simulink model "voitureAuto"  (R2019a)
settings: Solver=VariableStepAuto  StartTime=0.0  StopTime=5000  RelTol=1e-3
undefined symbols (not defined in the file or in its folder): BAT_AUTONOMY_KM, INIT_NIV_BAT, TIME_TO_CHARGE_S, VITESSE_MAX_KMH
libraries: simulink x2, simulink_extras x1, truetime x1
settings Model: SimulationMode=accelerator  Creator=PolyMTL  LastModifiedBy=angodb
settings DataIOCC: ReturnWorkspaceOutputs=off
settings OptimizationCC: EfficientMapNaN2IntZero=off
settings DebuggingCC: PregeneratedLibrarySubsystemCodeDiagnostic=none  ArithmeticOperatorsInVariantConditions=warning
settings HardwareCC: TargetBitPerPointer=64  TargetBitPerSizeT=64  TargetBitPerPtrDiffT=64  TargetLongLongMode=on  TargetIntDivRoundTo=Zero  TargetEndianess=LittleEndian  TargetWordSize=64  TargetHWDeviceType=MATLAB Host  ProdEqTarget=off
settings SFSimCC: SimUseLocalCustomCode=off
settings RTWCC: RTWUseLocalCustomCode=off
settings CodeAppCC: MaxIdLength=128
settings GRTTargetCC: TargetLangStandard=C89/C90 (ANSI)  CombineOutputUpdateFcns=off  GRTInterface=on

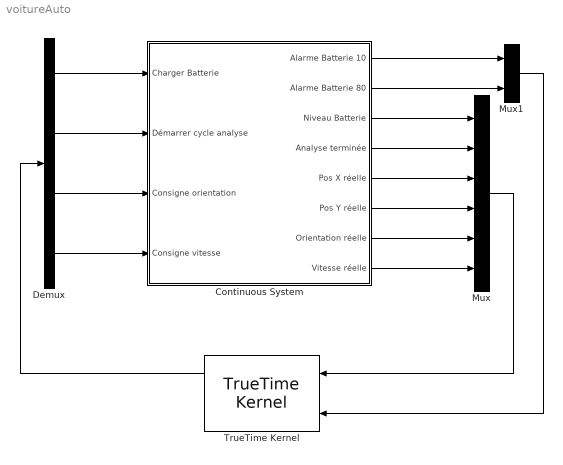
== system voitureAuto ==
  Continuous System : Subsystem
  Demux : Demux
  Mux : Mux  Inputs=6
  Mux1 : Mux  Inputs=2
  TrueTime Kernel : truetime/TrueTime Kernel  sfun=ctrlauto  args=[]  ninputsoutputs=[6 4]  ntriggers=2  trigtype=falling  nwnodenbr=[]  clockoffsetdrift=[0 0]  schedoutput=on  battery=off  poweroutput=off
  wires:
  Continuous System/5(Pos X réelle) -> Mux/3
  Continuous System/4(Analyse terminée) -> Mux/2
  Continuous System/3(Niveau Batterie) -> Mux/1
  Continuous System/8(Vitesse réelle) -> Mux/6
  Continuous System/7(Orientation réelle) -> Mux/5
  Continuous System/6(Pos Y réelle) -> Mux/4
  Demux/1 -> Continuous System/1(Charger Batterie)
  Demux/4 -> Continuous System/4(Consigne vitesse)
  Demux/3 -> Continuous System/3(Consigne orientation)
  Demux/2 -> Continuous System/2(Démarrer cycle analyse)
  Continuous System/1(Alarme Batterie 10) -> Mux1/1
  Continuous System/2(Alarme Batterie 80) -> Mux1/2
  Mux/1 -> TrueTime Kernel/1
  TrueTime Kernel/1 -> Demux/1
  Mux1/1 -> TrueTime Kernel/2

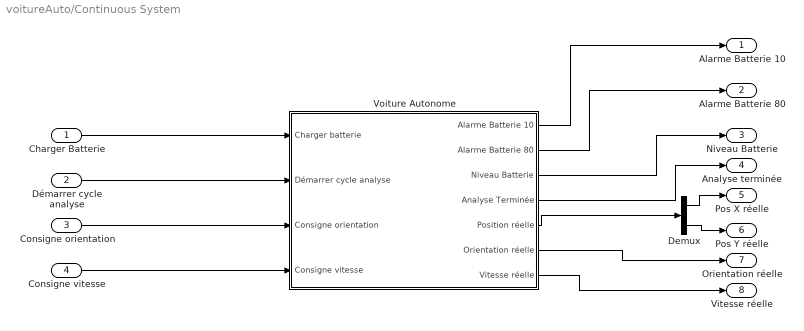
== system voitureAuto/Continuous System ==
  Charger Batterie : Inport
  Démarrer cycle analyse : Inport  Port=2
  Consigne orientation : Inport  Port=3
  Consigne vitesse : Inport  Port=4
  Demux : Demux  Outputs=2
  Voiture Autonome : Subsystem
  Alarme Batterie 10 : Outport
  Alarme Batterie 80 : Outport  Port=2
  Niveau Batterie : Outport  Port=3
  Analyse terminée : Outport  Port=4
  Pos X réelle : Outport  Port=5
  Pos Y réelle : Outport  Port=6
  Orientation réelle : Outport  Port=7
  Vitesse réelle : Outport  Port=8
  wires:
  Consigne orientation/1 -> Voiture Autonome/3(Consigne orientation)
  Démarrer cycle analyse/1 -> Voiture Autonome/2(Démarrer cycle analyse)
  Consigne vitesse/1 -> Voiture Autonome/4(Consigne vitesse)
  Voiture Autonome/3(Niveau Batterie) -> Niveau Batterie/1
  Voiture Autonome/1(Alarme Batterie 10) -> Alarme Batterie 10/1
  Voiture Autonome/4(Analyse Terminée) -> Analyse terminée/1
  Voiture Autonome/6(Orientation réelle) -> Orientation réelle/1
  Voiture Autonome/7(Vitesse réelle) -> Vitesse réelle/1
  Voiture Autonome/5(Position réelle) -> Demux/1
  Demux/1 -> Pos X réelle/1
  Demux/2 -> Pos Y réelle/1
  Charger Batterie/1 -> Voiture Autonome/1(Charger batterie)
  Voiture Autonome/2(Alarme Batterie 80) -> Alarme Batterie 80/1

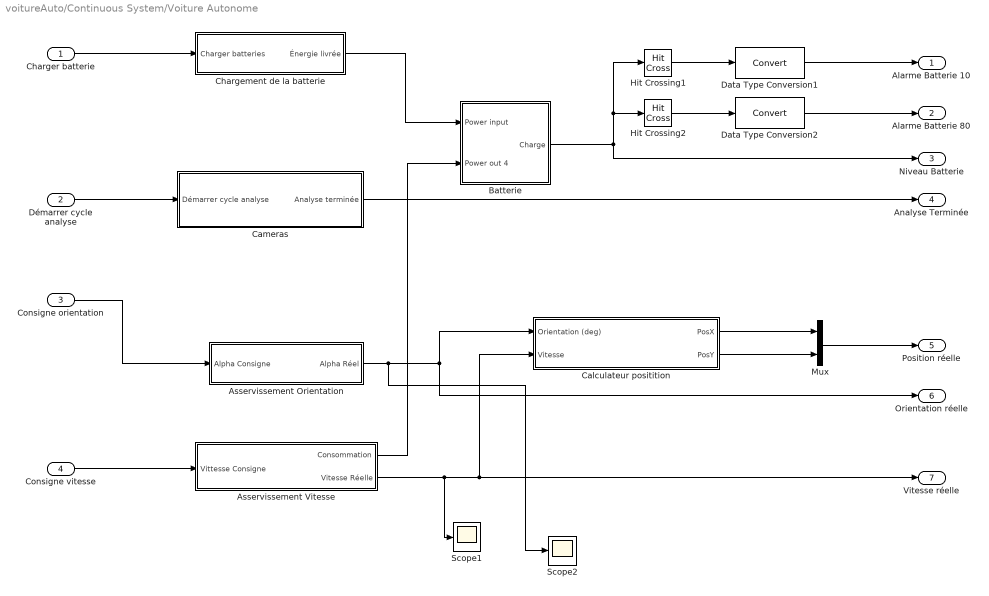
== system voitureAuto/Continuous System/Voiture Autonome ==
  Charger batterie : Inport
  Démarrer cycle analyse : Inport  Port=2
  Consigne orientation : Inport  Port=3
  Consigne vitesse : Inport  Port=4
  Asservissement Orientation : Subsystem
  Asservissement Vitesse : Subsystem
  Batterie : Subsystem
  Calculateur positition : Subsystem
  Cameras : Subsystem
  Chargement de la batterie : Subsystem
  Data Type Conversion1 : DataTypeConversion
  Data Type Conversion2 : DataTypeConversion
  Hit Crossing1 : HitCross  HitCrossingOffset=10  HitCrossingDirection=falling
  Hit Crossing2 : HitCross  HitCrossingOffset=80  HitCrossingDirection=rising
  Mux : Mux  Inputs=2
  Scope1 : Scope
  Scope2 : Scope
  Alarme Batterie 10 : Outport
  Alarme Batterie 80 : Outport  Port=2
  Niveau Batterie : Outport  Port=3
  Analyse Terminée : Outport  Port=4
  Position réelle : Outport  Port=5
  Orientation réelle : Outport  Port=6
  Vitesse réelle : Outport  Port=7
  wires:
  Hit Crossing1/1 -> Data Type Conversion1/1
  Data Type Conversion1/1 -> Alarme Batterie 10/1
  Asservissement Orientation/1(Alpha Réel) -> Scope2/1, Orientation réelle/1, Calculateur positition/1(Orientation (deg))
  Asservissement Vitesse/2(Vitesse Réelle) -> Calculateur positition/2(Vitesse), Vitesse réelle/1, Scope1/1
  Consigne orientation/1 -> Asservissement Orientation/1(Alpha Consigne)
  Mux/1 -> Position réelle/1
  Calculateur positition/2(PosY) -> Mux/2
  Calculateur positition/1(PosX) -> Mux/1
  Démarrer cycle analyse/1 -> Cameras/1(Démarrer cycle analyse)
  Cameras/1(Analyse terminée) -> Analyse Terminée/1
  Batterie/1(Charge) -> Hit Crossing1/1, Hit Crossing2/1, Niveau Batterie/1
  Chargement de la batterie/1(Énergie livrée) -> Batterie/1(Power input)
  Hit Crossing2/1 -> Data Type Conversion2/1
  Data Type Conversion2/1 -> Alarme Batterie 80/1
  Asservissement Vitesse/1(Consommation) -> Batterie/2(Power out 4)
  Charger batterie/1 -> Chargement de la batterie/1(Charger batteries)
  Consigne vitesse/1 -> Asservissement Vitesse/1(Vittesse Consigne)

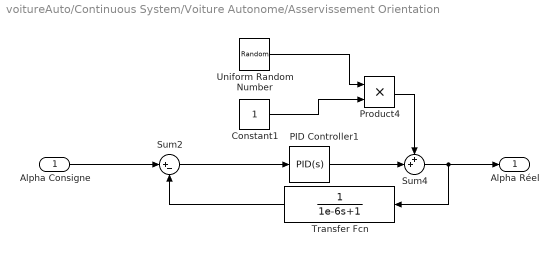
== system voitureAuto/Continuous System/Voiture Autonome/Asservissement Orientation ==
  Alpha Consigne : Inport
  Constant1 : Constant
  PID Controller1 : simulink/Continuous/PID Controller  Controller=PID  Form=Parallel  TimeDomain=Continuous-time  SampleTime=-1  IntegratorMethod=Forward Euler  FilterMethod=Forward Euler  ControllerParametersSource=internal  P=5  I=1  D=0  UseFilter=on  N=0.1  TunerSelectOption=Transfer Function Based (PID Tuner App)  InitialConditionSource=internal  InitialConditionForIntegrator=0  InitialConditionForFilter=0  DifferentiatorICPrevScaledInput=0  ExternalReset=none  TrackingMode=off  Kt=1  LimitOutput=off  UpperSaturationLimit=inf  LowerSaturationLimit=-inf  LinearizeAsGain=on  AntiWindupMode=none  Kb=1  POutMin=[]  POutMax=[]  IOutMin=[]  IOutMax=[]  DOutMin=[]  DOutMax=[]  NOutMin=[]  NOutMax=[]  SumOutMin=[]  SumOutMax=[]  SaturationOutMin=[]  SaturationOutMax=[]  PParamMin=[]  PParamMax=[]  IParamMin=[]  IParamMax=[]  DParamMin=[]  DParamMax=[]  NParamMin=[]  NParamMax=[]  KbParamMin=[]  KbParamMax=[]  KtParamMin=[]  KtParamMax=[]  KbOutMin=[]  KbOutMax=[]  KtOutMin=[]  KtOutMax=[]  IntegratorOutMin=[]  IntegratorOutMax=[]  FilterOutMin=[]  FilterOutMax=[]  SumI1OutMin=[]  SumI1OutMax=[]  SumI2OutMin=[]  SumI2OutMax=[]  SumI3OutMin=[]  SumI3OutMax=[]  SumI4OutMin=[]  SumI4OutMax=[]  SumDOutMin=[]  SumDOutMax=[]  DifferentiatorOutMin=[]  DifferentiatorOutMax=[]  FilterDiffOutCoefMin=[]  FilterDiffOutCoefMax=[]  ReciprocalOutMin=[]  ReciprocalOutMax=[]  SumDenOutMin=[]  SumDenOutMax=[]  SumNumOutMin=[]  SumNumOutMax=[]  DivideOutMin=[]  DivideOutMax=[]  IntegratorContinuousStateAttributes=''  IntegratorStateMustResolveToSignalObject=off  IntegratorRTWStateStorageClass=Auto  FilterContinuousStateAttributes=''  FilterStateMustResolveToSignalObject=off  FilterRTWStateStorageClass=Auto  ParallelPVariant=InternalParameters  IdealPVariant=Disabled  IVariant=InternalParameters  DVariant=InternalParameters  IntegratorVariant=Continuous  SatVariant=Disabled  AWVariant=Passthrough  PCopyVariant=Disabled  TRVariant=Disabled  FdbkBlocksVariant=Forward  IdealPFdbkVariant=Disabled  SatFdbkVariant=Disabled  DerivativeFilterVariant=ContFilter  NVariant=InternalParameters  NCopyVariant=Disabled  FilterICVariant=InternalICsFilter  IntegratorICVariant=InternalICs  ExternalResetVariant=Disabled  TRSumVariant=Passthrough  SumFdbkVariant=Disabled  SumVariant=Sum_PID
  Product4 : Product
  Sum2 : Sum  Inputs=|+-
  Sum4 : Sum  Inputs=++|
  Transfer Fcn : TransferFcn  Denominator=[1e-6 1]
  Uniform Random Number : UniformRandomNumber  SampleTime=0.1
  Alpha Réel : Outport
  wires:
  Product4/1 -> Sum4/1
  Uniform Random Number/1 -> Product4/1
  Alpha Consigne/1 -> Sum2/1
  Constant1/1 -> Product4/2
  Sum2/1 -> PID Controller1/1
  PID Controller1/1 -> Sum4/2
  Sum4/1 -> Transfer Fcn/1, Alpha Réel/1
  Transfer Fcn/1 -> Sum2/2

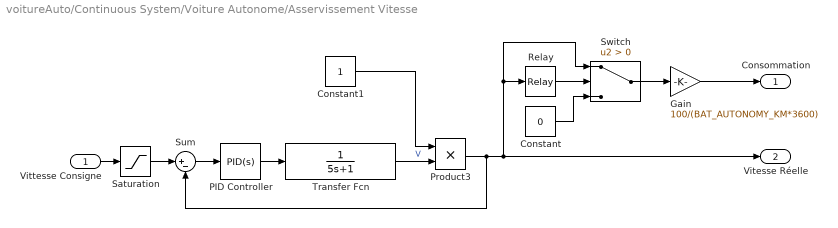
== system voitureAuto/Continuous System/Voiture Autonome/Asservissement Vitesse ==
  Vittesse Consigne : Inport
  Constant : Constant  Value=0
  Constant1 : Constant
  Gain : Gain  Gain=100/(BAT_AUTONOMY_KM*3600)
  PID Controller : simulink/Continuous/PID Controller  Controller=PID  Form=Parallel  TimeDomain=Continuous-time  SampleTime=-1  IntegratorMethod=Forward Euler  FilterMethod=Forward Euler  ControllerParametersSource=internal  P=2  I=0.5  D=0  UseFilter=on  N=0  TunerSelectOption=Transfer Function Based (PID Tuner App)  InitialConditionSource=internal  InitialConditionForIntegrator=0  InitialConditionForFilter=0  DifferentiatorICPrevScaledInput=0  ExternalReset=none  TrackingMode=off  Kt=1  LimitOutput=off  UpperSaturationLimit=inf  LowerSaturationLimit=-inf  LinearizeAsGain=on  AntiWindupMode=none  Kb=1  POutMin=[]  POutMax=[]  IOutMin=[]  IOutMax=[]  DOutMin=[]  DOutMax=[]  NOutMin=[]  NOutMax=[]  SumOutMin=[]  SumOutMax=[]  SaturationOutMin=[]  SaturationOutMax=[]  PParamMin=[]  PParamMax=[]  IParamMin=[]  IParamMax=[]  DParamMin=[]  DParamMax=[]  NParamMin=[]  NParamMax=[]  KbParamMin=[]  KbParamMax=[]  KtParamMin=[]  KtParamMax=[]  KbOutMin=[]  KbOutMax=[]  KtOutMin=[]  KtOutMax=[]  IntegratorOutMin=[]  IntegratorOutMax=[]  FilterOutMin=[]  FilterOutMax=[]  SumI1OutMin=[]  SumI1OutMax=[]  SumI2OutMin=[]  SumI2OutMax=[]  SumI3OutMin=[]  SumI3OutMax=[]  SumI4OutMin=[]  SumI4OutMax=[]  SumDOutMin=[]  SumDOutMax=[]  DifferentiatorOutMin=[]  DifferentiatorOutMax=[]  FilterDiffOutCoefMin=[]  FilterDiffOutCoefMax=[]  ReciprocalOutMin=[]  ReciprocalOutMax=[]  SumDenOutMin=[]  SumDenOutMax=[]  SumNumOutMin=[]  SumNumOutMax=[]  DivideOutMin=[]  DivideOutMax=[]  IntegratorContinuousStateAttributes=''  IntegratorStateMustResolveToSignalObject=off  IntegratorRTWStateStorageClass=Auto  FilterContinuousStateAttributes=''  FilterStateMustResolveToSignalObject=off  FilterRTWStateStorageClass=Auto  ParallelPVariant=InternalParameters  IdealPVariant=Disabled  IVariant=InternalParameters  DVariant=InternalParameters  IntegratorVariant=Continuous  SatVariant=Disabled  AWVariant=Passthrough  PCopyVariant=Disabled  TRVariant=Disabled  FdbkBlocksVariant=Forward  IdealPFdbkVariant=Disabled  SatFdbkVariant=Disabled  DerivativeFilterVariant=ContFilter  NVariant=InternalParameters  NCopyVariant=Disabled  FilterICVariant=InternalICsFilter  IntegratorICVariant=InternalICs  ExternalResetVariant=Disabled  TRSumVariant=Passthrough  SumFdbkVariant=Disabled  SumVariant=Sum_PID
  Product3 : Product
  Relay : Relay  OnSwitchValue=0.051  OffSwitchValue=0.05
  Saturation : Saturate  UpperLimit=VITESSE_MAX_KMH  LowerLimit=0
  Sum : Sum  Inputs=|+-
  Switch : Switch  Criteria=u2 > Threshold
  Transfer Fcn : TransferFcn  Denominator=[5 1]
  Consommation : Outport
  Vitesse Réelle : Outport  Port=2
  wires:
  Vittesse Consigne/1 -> Saturation/1
  Transfer Fcn/1 -> Product3/2  "V"
  Product3/1 -> Switch/1, Relay/1, Vitesse Réelle/1, Sum/2
  Relay/1 -> Switch/2
  Gain/1 -> Consommation/1
  Saturation/1 -> Sum/1
  Switch/1 -> Gain/1
  Constant/1 -> Switch/3
  Sum/1 -> PID Controller/1
  PID Controller/1 -> Transfer Fcn/1
  Constant1/1 -> Product3/1

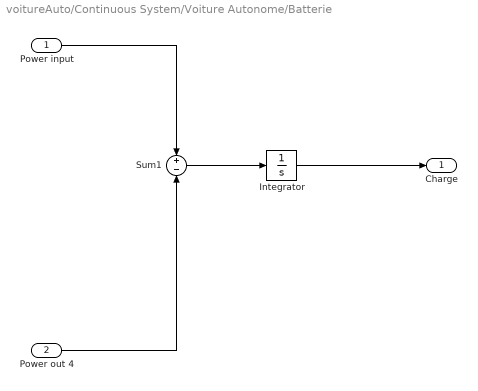
== system voitureAuto/Continuous System/Voiture Autonome/Batterie ==
  Power input : Inport
  Power out 4 : Inport  Port=2
  Integrator : Integrator  InitialCondition=INIT_NIV_BAT  LimitOutput=on  UpperSaturationLimit=100  LowerSaturationLimit=0
  Sum1 : Sum  Inputs=+-
  Charge : Outport
  wires:
  Sum1/1 -> Integrator/1
  Power input/1 -> Sum1/1
  Power out 4/1 -> Sum1/2
  Integrator/1 -> Charge/1

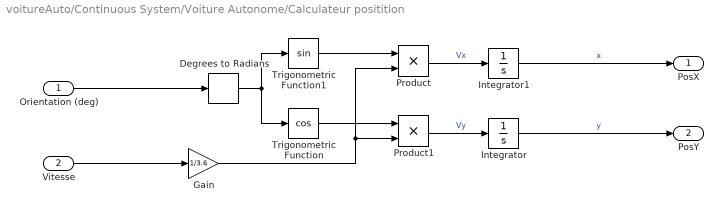
== system voitureAuto/Continuous System/Voiture Autonome/Calculateur positition ==
  Orientation (deg) : Inport
  Vitesse : Inport  Port=2
  Degrees to Radians : simulink_extras/Transformations/Degrees to Radians
  Gain : Gain  Gain=1/3.6
  Integrator : Integrator
  Integrator1 : Integrator
  Product : Product
  Product1 : Product
  Trigonometric Function : Trigonometry  Operator=cos
  Trigonometric Function1 : Trigonometry
  PosX : Outport
  PosY : Outport  Port=2
  wires:
  Integrator/1 -> PosY/1  "y"
  Product/1 -> Integrator1/1  "Vx"
  Trigonometric Function1/1 -> Product/1
  Degrees to Radians/1 -> Trigonometric Function1/1, Trigonometric Function/1
  Trigonometric Function/1 -> Product1/1
  Product1/1 -> Integrator/1  "Vy"
  Integrator1/1 -> PosX/1  "x"
  Vitesse/1 -> Gain/1
  Orientation (deg)/1 -> Degrees to Radians/1
  Gain/1 -> Product/2, Product1/2

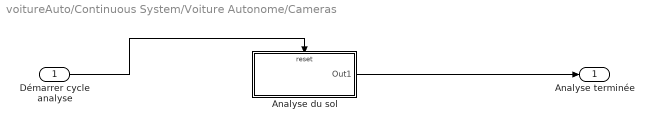
== system voitureAuto/Continuous System/Voiture Autonome/Cameras ==
  Démarrer cycle analyse : Inport
  Analyse du sol : Subsystem  TreatAsAtomicUnit=on
  Analyse terminée : Outport
  wires:
  Démarrer cycle analyse/1 -> Analyse du sol/Reset
  Analyse du sol/1(Out1) -> Analyse terminée/1

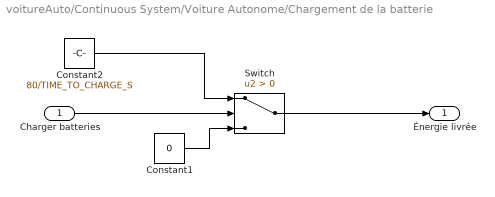
== system voitureAuto/Continuous System/Voiture Autonome/Chargement de la batterie ==
  Charger batteries : Inport
  Constant1 : Constant  Value=0
  Constant2 : Constant  Value=80/TIME_TO_CHARGE_S
  Switch : Switch  Criteria=u2 > Threshold
  Énergie livrée : Outport
  wires:
  Charger batteries/1 -> Switch/2
  Constant1/1 -> Switch/3
  Switch/1 -> Énergie livrée/1
  Constant2/1 -> Switch/1

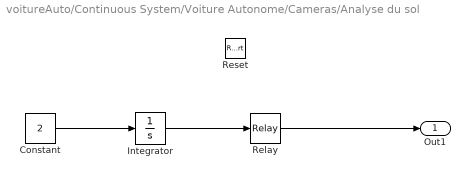
== system voitureAuto/Continuous System/Voiture Autonome/Cameras/Analyse du sol ==
  Reset : ResetPort  DisableCoverage=on
  Constant : Constant  Value=2
  Integrator : Integrator
  Relay : Relay  OnSwitchValue=1  OffSwitchValue=0
  Out1 : Outport
  wires:
  Integrator/1 -> Relay/1
  Constant/1 -> Integrator/1
  Relay/1 -> Out1/1
